simulink library "lib_controls2"  (Simulink 10.1)
settings: Solver=VariableStepAuto  StartTime=0.0  StopTime=10.0  RelTol=1e-3
undefined symbols (not defined in the file or in its folder): cs_charge_deplete_bool, cs_charge_pwr, cs_charge_trq, cs_fc_init_state, cs_hi_soc, cs_lo_soc, cs_max_pwr, cs_max_pwr_fall_rate, cs_max_pwr_rise_rate, cs_min_off_time, cs_min_pwr, cs_min_trq_frac, cs_pwr, cs_spd, ess_on, fc_map_spd, fc_max_trq, fc_on, fc_spd_scale, fc_trq_scale, gc_map_spd, gc_map_trq, gc_outpwr_map, gc_spd_scale, gc_trq_scale
settings Model: Creator=sateeshk  LastModifiedBy=sateeshk
settings Model: ModifiedComment=|
  | bjeanner -- Thu Dec 26 09:42:29 2002 -- Version 1.451
  | add three new parameters: allowing calcultion of equivallent ESS function with mean efficiency; plus plotting results parameter
settings Model: ModifiedHistory=|
  | bjeanner -- Thu Dec 26 09:42:29 2002 -- Version 1.451
  | add three new parameters: allowing calcultion of equivallent ESS function with mean efficiency; plus plotting results parameter
  | 
  | 
  | bjeanner -- Thu Dec 26 09:42:29 2002 -- Version 1.451
  | add three new parameters: allowing calcultion of equivallent ESS function with mean efficiency; plus plotting results parameter
  | 
  | 
  | bjeanner -- Thu Dec 12 14:52:52 2002 -- Version 1.450
  | 
  | 
  | bjeanner -- Tue Dec 10 14:49:05 2002 -- Version 1.449
  | 
  | 
  | bjeanner -- Tue Dec 10 13:14:31 2002 -- Version 1.448
  | 
  | 
  | bjeanner -- Tue Dec 10 11:50:56 2002 -- Version 1.447
  | 
  | 
  | bjeanner -- Tue Dec 10 11:41:01 2002 -- Version 1.446
  | 
  | 
  | bjeanner -- Tue Dec 10 11:30:40 2002 -- Version 1.445
  | 
  | 
  | bjeanner -- Tue Dec 10 11:29:40 2002 -- Version 1.444
  | 
  | 
  | bjeanner -- Tue Dec 10 11:10:40 2002 -- Version 1.443
  | 
  | 
  | bjeanner -- Tue Dec 10 10:31:25 2002 -- Version 1.442
  | 
  | 
  | bjeanner -- Tue Dec 10 10:30:04 2002 -- Version 1.441
  | 
  | 
  | bjeanner -- Tue Dec 10 10:29:36 2002 -- Version 1.440
  | 
  | 
  | bjeanner -- Tue Dec 10 10:23:30 2002 -- Version 1.439
  | 
  | 
  | bjeanner -- Tue Dec 10 09:20:40 2002 -- Version 1.438
  | 
  | 
  | bjeanner -- Tue Dec 10 09:16:26 2002 -- Version 1.437
  | Add the template for the configurable subsystem for the BD_FUELCELL control strategy.
  | Add the fuel cell adaptive control strategy
  | 
  | 
  | mokeefe -- Tue Aug 13 07:36:17 2002 -- Version 1.436
  | Making the model look "pretty"
  | 
  | mokeefe -- Tue Aug 13 07:35:11 2002 -- Version 1.435
  | changed <vc> conv cvt/cvt control to use "acc_mech_pwr_est" instead of "acc_mech_trq_est" as had been used previously (the required datum is the power and not the torque!)
  | 
  | ssprik -- Tue Apr 30 11:21:35 2002 -- Version 1.434
  | added user contributed par bal engine on  block
  | 
  | mokeefe -- Tue Apr 23 09:06:10 2002 -- Version 1.433
  | changed Insight electric assist control strategy <cs> DIRECT SPLIT/Hard Acceleration to prevent a divide by zero warning. Also added logic to prevent a torque request above the maximum achievable motor torque.
  | 
  | mokeefe -- Tue Apr 23 09:03:51 2002 -- Version 1.432
  | changed Insight electric assist control strategy <cs> DIRECT SPLIT/Hard Acceleration to prevent a divide by zero warning. Also added logic to prevent a torque request above the maximum achievable motor torque.
  | 
  | mokeefe -- Tue Apr 23 08:50:58 2002 -- Version 1.431
  | 
  | 
  | ssprik -- Thu Apr 18 14:34:50 2002 -- Version 1.430
  | 
  | 
  | ssprik -- Thu Apr 18 14:32:52 2002 -- Version 1.429
  | 
  | 
  | ssprik -- Thu Apr 18 14:06:57 2002 -- Version 1.428
  | 
  | 
  | ssprik -- Thu Apr 18 13:56:10 2002 -- Version 1.427
  | 
  | 
  | ssprik -- Thu Apr 18 13:46:32 2002 -- Version 1.426
  | 
  | 
  | kkelly -- Thu Apr 18 10:17:40 2002 -- Version 1.425
  | 
  | 
  | mokeefe -- Thu Apr 18 08:23:32 2002 -- Version 1.424
  | saving the model:
  | o "without the model browser open"
  | o with only top-level screen visible
  | o with "fit to view" enabled
  | o with "status bar" off and "toolbar" off
  | o with "prompt to update model history with each save" on
  | 
  | kkelly -- Wed Mar 27 14:57:12 2002 -- Version 1.423
  | 
  | 
  | kkelly -- Wed Mar 27 14:57:12 2002 -- Version 1.423
  | 
  | 
  | kkelly -- Wed Mar 27 14:50:41 2002 -- Version 1.422
  | 
  | 
  | kkelly -- Wed Mar 27 14:50:24 2002 -- Version 1.421
  | 
  | 
  | kkelly -- Wed Mar 27 14:26:31 2002 -- Version 1.420
  | 
  | 
  | kkelly -- Wed Mar 27 14:26:16 2002 -- Version 1.419
  | 
  | 
  | kkelly -- Wed Mar 27 14:25:54 2002 -- Version 1.418
  | 
  | 
  | kkelly -- Wed Mar 27 14:20:49 2002 -- Version 1.417
  | 
  | 
  | kkelly -- Wed Mar 27 14:18:25 2002 -- Version 1.416
  | 
  | 
  | kkelly -- Wed Mar 27 14:17:14 2002 -- Version 1.415
  | 
  | 
  | kkelly -- Wed Mar 27 14:09:18 2002 -- Version 1.414
  | 
  | 
  | kkelly -- Wed Mar 27 14:07:10 2002 -- Version 1.413
  | 
  | 
  | kkelly -- Wed Mar 27 14:04:42 2002 -- Version 1.412
  | 
  | 
  | kkelly -- Wed Mar 27 12:39:55 2002 -- Version 1.411
  | 
  | 
  | kkelly -- Wed Mar 27 12:39:35 2002 -- Version 1.410
  | 
  | 
  | kkelly -- Wed Mar 27 12:31:18 2002 -- Version 1.409
  | 
  | 
  | kkelly -- Wed Mar 27 12:12:25 2002 -- Version 1.408
  | 
  | 
  | kkelly -- Wed Mar 27 12:03:57 2002 -- Version 1.407
  | 
  | 
  | kkelly -- Wed Mar 27 12:03:11 2002 -- Version 1.406
  | Added logic to increase torque request for very hard acceleration
  | 
  | kkelly -- Wed Mar 27 11:51:32 2002 -- Version 1.405
  | Added logic to allow EM in 1st gear when torque request is high
  | 
  | kkelly -- Wed Mar 27 11:48:18 2002 -- Version 1.404
  | Added logic to allow EM at low speed with high torque request
  | 
  | kkelly -- Wed Mar 27 11:36:20 2002 -- Version 1.403
  | Added zero-torque request logic
  | 
  | kkelly -- Wed Mar 27 11:09:35 2002 -- Version 1.402
  | 
  | 
  | kkelly -- Wed Mar 27 11:07:39 2002 -- Version 1.401
  | 
  | 
  | kkelly -- Wed Mar 27 10:43:33 2002 -- Version 1.400
  | 
  | 
  | mokeefe -- Fri Mar 08 08:11:28 2002 -- Version 1.399
  | took all separate auxiliary load calculations out of the <vc> libraries. These will now use the lib_accessory goto tags (acc_mech_trq_est, acc_mech_pwr_est, acc_elec_pwr_est)
  | 
  | mokeefe -- Mon Jul 02 10:08:55 2001 -- Version 1.184
  | 
  | 
  | mokeefe -- Mon Jul 02 10:08:07 2001 -- Version 1.183
  | 
  | 
  | mokeefe -- Mon Jul 02 10:06:51 2001 -- Version 1.182
  | 
  | 
  | mokeefe -- Mon Jul 02 10:05:17 2001 -- Version 1.181
  | 
  | 
  | mokeefe -- Mon Jul 02 10:04:17 2001 -- Version 1.180
  | 
  | 
  | mokeefe -- Fri Jun 29 13:59:18 2001 -- Version 1.179
  | 
  | all <vc> blocks updated for use with variable cargo mass functionality (cargo mass by distance)--also, all <vc> top-level blocks have been "cleaned up" to look neat and organized. A sub-model library has been made and is the preferred way to do future development.
  | 
  | mokeefe -- Fri Jun 29 13:56:37 2001 -- Version 1.178
  | 
  | <vc> prius
  | 
  | mokeefe -- Fri Jun 29 13:46:29 2001 -- Version 1.177
  | 
  | 
  | mokeefe -- Fri Jun 29 13:40:43 2001 -- Version 1.176
  | 
  | 
  | mokeefe -- Fri Jun 29 13:39:38 2001 -- Version 1.175
  | 
  | <vc> series ("" "")
  | 
  | 
  | mokeefe -- Fri Jun 29 13:34:00 2001 -- Version 1.174
  | 
  | <vc> par Adaptive ("" "")
  | 
  | mokeefe -- Fri Jun 29 13:23:41 2001 -- Version 1.173
  | 
  | insight (ibid.)
  | 
  | 
  | mokeefe -- Fri Jun 29 13:15:22 2001 -- Version 1.172
  | 
  | <vc> par balanced--> veh_mass to veh_mass+veh_cargo_mass
  | 
  | 
  | mokeefe -- Fri Jun 29 13:05:39 2001 -- Version 1.171
  | 
  | 
  | mokeefe -- Fri Jun 29 12:10:12 2001 -- Version 1.170
  | 
  | finished veh_mass mods for the <vc> par cvt...
  | 
  | 
  | mokeefe -- Fri Jun 29 12:09:18 2001 -- Version 1.169
  | 
  | 
  | mokeefe -- Fri Jun 29 11:56:20 2001 -- Version 1.168
  | 
  | 
  | mokeefe -- Fri Jun 29 11:44:30 2001 -- Version 1.167
  | 
  | 
  | mokeefe -- Fri Jun 29 11:33:07 2001 -- Version 1.166
  | 
  | 
  | mokeefe -- Fri Jun 29 11:21:54 2001 -- Version 1.165
  | 
  | 
  | mokeefe -- Fri Jun 29 11:15:04 2001 -- Version 1.164
  | 
  | 
  | mokeefe -- Fri Jun 29 11:13:02 2001 -- Version 1.163
  | 
  | 
  | mokeefe -- Fri Jun 29 11:06:47 2001 -- Version 1.162
  | 
  | 
  | mokeefe -- Fri Jun 29 11:04:27 2001 -- Version 1.161
  | 
  | 
  | mokeefe -- Fri Jun 29 10:40:33 2001 -- Version 1.160
  | 
  | 
  | mokeefe -- Fri Jun 29 10:35:18 2001 -- Version 1.159
  | 
  | 
  | mokeefe -- Fri Jun 29 10:29:06 2001 -- Version 1.158
  | 
  | 
  | mokeefe -- Fri Jun 29 10:26:50 2001 -- Version 1.157
  | 
  | 
  | mokeefe -- Fri Jun 29 10:18:10 2001 -- Version 1.156
  | 
  | made traction control, front and rear brake controller, and braking strategy into "sub-libraries" for vehicle control
  | 
  | mokeefe -- Fri Jun 29 10:17:11 2001 -- Version 1.155
  | 
  | 
  | mokeefe -- Fri Jun 29 10:15:46 2001 -- Version 1.154
  | 
  | 
  | mokeefe -- Fri Jun 29 10:09:48 2001 -- Version 1.153
  | 
  | 
  | mokeefe -- Fri Jun 29 09:58:42 2001 -- Version 1.152
  | 
  | 
  | mokeefe -- Fri Jun 29 09:57:37 2001 -- Version 1.151
  | 
  | creating sub-components for vehicle control model (traction control)
  | 
  | mokeefe -- Fri Jun 29 09:21:23 2001 -- Version 1.150
  | 
  | 
  | mokeefe -- Fri Jun 29 09:19:46 2001 -- Version 1.149
  | 
  | 
  | mokeefe -- Fri Jun 29 09:09:49 2001 -- Version 1.148
  | 
  | 
  | mokeefe -- Fri Jun 29 08:32:46 2001 -- Version 1.147
  | 
  | 
  | mokeefe -- Fri Jun 29 08:29:03 2001 -- Version 1.146
  | 
  | replacing veh_mass with veh_mass plus veh_cargo_mass in <vc> conv auto Saber Custom
  | 
  | 
  | mokeefe -- Thu Jun 28 17:08:40 2001 -- Version 1.145
  | 
  | 
  | mokeefe -- Thu Jun 28 17:07:02 2001 -- Version 1.144
  | 
  | 
  | mokeefe -- Thu Jun 28 17:06:28 2001 -- Version 1.143
  | 
  | changes to the CVT controls to subsitute veh_mass + veh_cargo_mass for veh_mass
  | 
  | 
  | mokeefe -- Thu Jun 28 16:55:42 2001 -- Version 1.142
  | 
  | 
  | mokeefe -- Thu Jun 28 16:32:01 2001 -- Version 1.141
  | 
  | changing veh_mass to veh_mass plus veh_cargo_mass
  | 
  | 
  | mokeefe -- Thu Jun 28 16:21:30 2001 -- Version 1.140
  | 
  | replacing veh_mass with veh_mass + (cargo mass vs time)
  | 
  | mokeefe -- Thu Jun 28 14:12:51 2001 -- Version 1.139
  | 
  | replaced all 'veh_mass' references with a veh_mass plus a FROM block (originating from drive cycle) that gives variable cargo mass by time

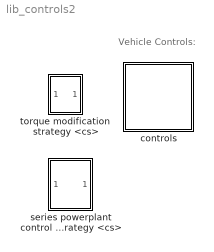
== system lib_controls2 ==
  note: Vehicle Controls:
  controls : Subsystem
  series powerplant control strategy <cs> : Subsystem  mask(Stand-Alone Series Powerplant Control Strategy Mask){generalName='cs', logPick=Log, initFileName={}, modCell={}, imgFileName='bdi_cs.jpg', DEBUG=OFF}
      mask prompts: generalName "General Name of this Component [char]"; logPick "Log Variables to Workspace?"; initFileName "Initialization File(s) [cell array of char]"; modCell "Modification Cell [2 column cell array of param and val]"; imgFileName "Icon image file name [char--evaluated]"
      mask init:
      | % initialization via m-file script
      | advSACompMaskInit;
      mask TypeOptions logPick: Don't Log | Log
      mask TypeOptions DEBUG: ON | OFF
      mask Display: image(imread(imgFileName))
  torque modification  strategy <cs> : Subsystem  mask(Stand-Alone Torque Modification Strategy Mask){generalName='tm', logPick=Log, initFileName={}, modCell={}, imgFileName='bdi_hybrid_cntrl.jpg', DEBUG=OFF}
      mask prompts: generalName "General Name of this Component [char]"; logPick "Log Variables to Workspace?"; initFileName "Initialization File(s) [cell array of char]"; modCell "Modification Cell [2 column cell array of param and val]"; imgFileName "Icon image file name [char--evaluated]"
      mask init:
      | % initialization via m-file script
      | advSACompMaskInit;
      mask TypeOptions logPick: Don't Log | Log
      mask TypeOptions DEBUG: ON | OFF
      mask Display: image(imread(imgFileName))

== system lib_controls2/controls ==
  Hybrid  Engine Torque Modification Strategy : Subsystem
      mask Display: image(imread('bdi_hybrid_cntrl.jpg'))

== system lib_controls2/series powerplant control strategy <cs> ==
  note: Series Powerplant Control Strategy
  power req'd by bus (W) : Inport
  Model and Interface : Subsystem
  power follower : Subsystem
      settings: OpenFcn=web(['file:\\\' which('Series.htm')]);
      mask Display: image(imread('doc_man.jpg'))
  thermostat : Subsystem
      settings: OpenFcn=web(['file:\\\' which('Series-therm.htm')]);
      mask Display: image(imread('doc_man.jpg'))
  "engine torque and speed (Nm), (rad/s)" : Outport  InitialOutput=0
  tag scope: csReqOut=global, csSensors=global
  wires:
  Model and Interface/2("engine torque and speed (Nm), (rad/s)") -> "engine torque and speed (Nm), (rad/s)"/1
  power req'd by bus (W)/1 -> Model and Interface/1(power req'd by bus (W))
  Model and Interface/1(req'd out) -> [csReqOut]
  [csControl] -> Model and Interface/2(control)
  Model and Interface/3(sensors) -> [csSensors]

== system lib_controls2/torque modification  strategy <cs> ==
  note: Torque Modification Strategy
  "original torque and speed req'd (Nm), (rad/s)" : Inport
  Block NOTES : Subsystem
      mask Display: disp('Block\nNOTES')
  help1 : Subsystem
      settings: OpenFcn=web(['file:\\\' which('cs_tips.htm')]);
      mask Display: image(imread('doc_man.jpg'))
  torque mod  model & interface : Subsystem
  "modified torque and speed req'd (Nm), (rad/s)" : Outport  InitialOutput=0
  tag scope: tmReqOut=global, tmSensors=global
  wires:
  torque mod  model & interface/3(sensors) -> [tmSensors]
  [tmControl] -> torque mod  model & interface/2(controls)
  "original torque and speed req'd (Nm), (rad/s)"/1 -> torque mod  model & interface/1(trq and spd output request)
  torque mod  model & interface/2(trq and spd input request) -> "modified torque and speed req'd (Nm), (rad/s)"/1
  torque mod  model & interface/1(requested output) -> [tmReqOut]

== system lib_controls2/controls/Hybrid  Engine Torque Modification Strategy ==
  Bus Creator : BusCreator  Inputs=3
  Bus Selector : BusSelector  OutputSignals=tm_spd_out_r
  Bus Selector1 : BusSelector  OutputSignals=SOC
  Bus Selector2 : BusSelector  OutputSignals=engine_on
  parallel auto hybrid torque control : Subsystem
  tag scope: tmControl=global
  wires:
  parallel auto hybrid torque control/1(tm_torqueMod) -> Bus Creator/1  "tm_torqueMod"
  parallel auto hybrid torque control/2(tm_torqueMin) -> Bus Creator/2  "tm_torqueMin"
  parallel auto hybrid torque control/3(tm_enable) -> Bus Creator/3  "tm_enable"
  Bus Creator/1 -> [tmControl]
  [tmReqOut] -> Bus Selector/1
  Bus Selector/1 -> parallel auto hybrid torque control/1(tm_spd_out_r)  "<tm_spd_out_r>"
  [essSensors] -> Bus Selector1/1
  Bus Selector1/1 -> parallel auto hybrid torque control/2(SOC)  "<SOC>"
  [fcControl] -> Bus Selector2/1
  Bus Selector2/1 -> parallel auto hybrid torque control/3(engine_on)  "<engine_on>"

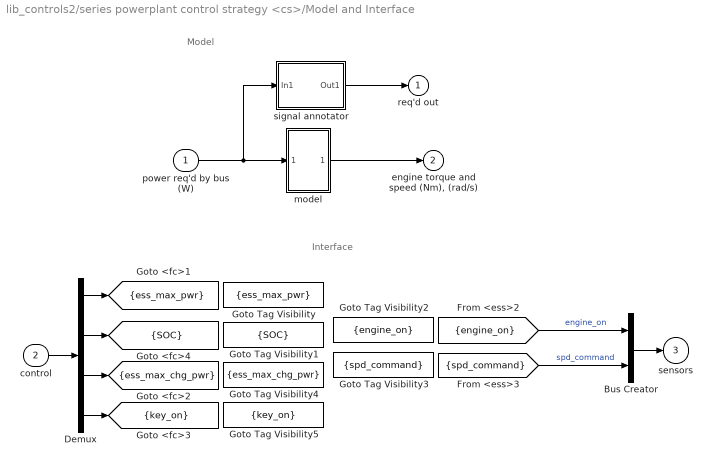
== system lib_controls2/series powerplant control strategy <cs>/Model and Interface ==
  note: Interface
  note: Model
  power req'd by bus (W) : Inport
  control : Inport  Port=2
  Bus Creator : BusCreator  Inputs=2
  Demux : Demux
  Goto Tag Visibility : GotoTagVisibility  GotoTag=ess_max_pwr
  Goto Tag Visibility1 : GotoTagVisibility  GotoTag=SOC
  Goto Tag Visibility2 : GotoTagVisibility  GotoTag=engine_on
  Goto Tag Visibility3 : GotoTagVisibility  GotoTag=spd_command
  Goto Tag Visibility4 : GotoTagVisibility  GotoTag=ess_max_chg_pwr
  Goto Tag Visibility5 : GotoTagVisibility  GotoTag=key_on
  model : Subsystem
  signal annotator : Subsystem
  req'd out : Outport  InitialOutput=0
  "engine torque and speed (Nm), (rad/s)" : Outport  Port=2  InitialOutput=0
  sensors : Outport  Port=3  InitialOutput=0
  tag scope: SOC=scoped, ess_max_chg_pwr=scoped, ess_max_pwr=scoped, key_on=scoped
  wires:
  model/1(Out1) -> "engine torque and speed (Nm), (rad/s)"/1
  power req'd by bus (W)/1 -> model/1(In1), signal annotator/1(In1)
  signal annotator/1(Out1) -> req'd out/1
  control/1 -> Demux/1
  Demux/1 -> [ess_max_pwr]
  Demux/2 -> [SOC]
  Demux/3 -> [ess_max_chg_pwr]
  Demux/4 -> [key_on]
  Bus Creator/1 -> sensors/1
  [engine_on] -> Bus Creator/1  "engine_on"
  [spd_command] -> Bus Creator/2  "spd_command"

== system lib_controls2/series powerplant control strategy <cs>/power follower ==

== system lib_controls2/series powerplant control strategy <cs>/thermostat ==

== system lib_controls2/torque modification  strategy <cs>/Block NOTES ==
  note: This model allows for increasing or decreasing of torque along a connection for purposes
      | of hybrid charging and control strategy.

== system lib_controls2/torque modification  strategy <cs>/help1 ==

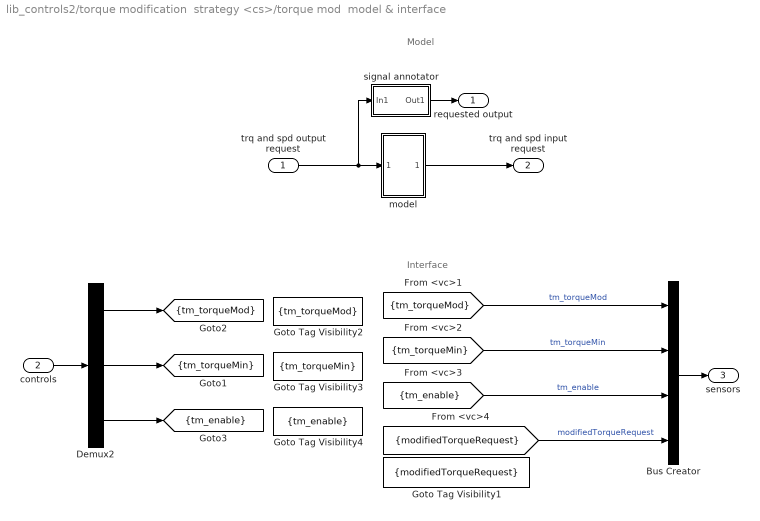
== system lib_controls2/torque modification  strategy <cs>/torque mod  model & interface ==
  note: Interface
  note: Model
  trq and spd output request : Inport
  controls : Inport  Port=2
  Bus Creator : BusCreator  Inputs=4
  Demux2 : Demux  Outputs=3
  Goto Tag Visibility1 : GotoTagVisibility  GotoTag=modifiedTorqueRequest
  Goto Tag Visibility2 : GotoTagVisibility  GotoTag=tm_torqueMod
  Goto Tag Visibility3 : GotoTagVisibility  GotoTag=tm_torqueMin
  Goto Tag Visibility4 : GotoTagVisibility  GotoTag=tm_enable
  model : Subsystem
  signal annotator : Subsystem
  requested output : Outport
  trq and spd input request : Outport  Port=2
  sensors : Outport  Port=3
  tag scope: tm_enable=scoped, tm_torqueMin=scoped, tm_torqueMod=scoped
  wires:
  signal annotator/1(Out1) -> requested output/1
  model/1(T,w modified) -> trq and spd input request/1
  trq and spd output request/1 -> signal annotator/1(In1), model/1("T, w original")
  Demux2/1 -> [tm_torqueMod]
  controls/1 -> Demux2/1
  Bus Creator/1 -> sensors/1
  [tm_torqueMod] -> Bus Creator/1  "tm_torqueMod"
  Demux2/2 -> [tm_torqueMin]
  Demux2/3 -> [tm_enable]
  [tm_torqueMin] -> Bus Creator/2  "tm_torqueMin"
  [tm_enable] -> Bus Creator/3  "tm_enable"
  [modifiedTorqueRequest] -> Bus Creator/4  "modifiedTorqueRequest"

== system lib_controls2/controls/Hybrid  Engine Torque Modification Strategy/parallel auto hybrid torque control ==
  tm_spd_out_r : Inport
  SOC : Inport  Port=2
  engine_on : Inport  Port=3
  chg trq req'd (Nm) : Subsystem
  minimum trq (Nm) : Subsystem
  tm_torqueMod : Outport
  tm_torqueMin : Outport  Port=2
  tm_enable : Outport  Port=3
  wires:
  tm_spd_out_r/1 -> minimum trq (Nm)/1("spd req'd in (N*m, rad/s)")
  SOC/1 -> minimum trq (Nm)/2(SOC), chg trq req'd (Nm)/1(SOC)
  minimum trq (Nm)/1(minimum trq (N*m)) -> tm_torqueMin/1
  engine_on/1 -> tm_enable/1
  chg trq req'd (Nm)/1(add'l trq req'd (Nm)) -> tm_torqueMod/1

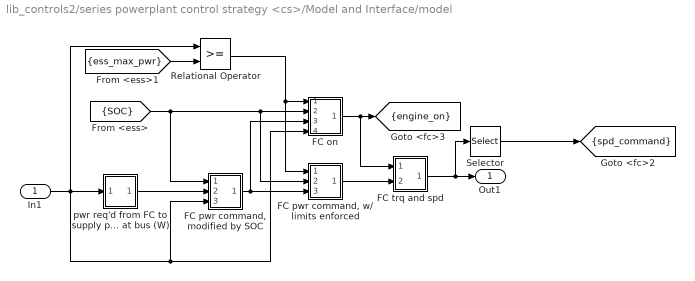
== system lib_controls2/series powerplant control strategy <cs>/Model and Interface/model ==
  In1 : Inport
  FC on : Subsystem
  "FC pwr command, modified by SOC" : Subsystem
  "FC pwr command, w/ limits enforced" : Subsystem
  FC trq and spd : Subsystem
  Relational Operator : RelationalOperator  RndMeth=Nearest  InputSameDT=on
  Selector : Selector  InputPortWidth=2  IndexOptions=Index vector (dialog)  Indices=2  OutputSizes=1
  pwr req'd from FC to supply pwr req'd at bus (W) : Subsystem
  Out1 : Outport
  tag scope: engine_on=scoped, spd_command=scoped
  wires:
  [SOC] -> "FC pwr command, modified by SOC"/1(SOC), "FC pwr command, w/ limits enforced"/2(SOC), FC on/2(SOC)
  "FC pwr command, modified by SOC"/1(pwr command modifed for SOC (W)) -> FC on/3(FC pwr command), "FC pwr command, w/ limits enforced"/3(FC pwr command)
  pwr req'd from FC to supply pwr req'd at bus (W)/1(pwr req'd of FC (W)) -> "FC pwr command, modified by SOC"/2(raw pwr command (W))
  Relational Operator/1 -> "FC pwr command, w/ limits enforced"/1(ess max pwr would be insufficient), FC on/1(ess max pwr would be insufficient)
  [ess_max_pwr] -> Relational Operator/2
  In1/1 -> pwr req'd from FC to supply pwr req'd at bus (W)/1(power req'd by bus (W)), Relational Operator/1, "FC pwr command, modified by SOC"/3(pwr req'd at bus (W)), FC on/4(bus pwr req)
  FC on/1(FC on) -> FC trq and spd/1(FC on), [engine_on]
  "FC pwr command, w/ limits enforced"/1(limited FC pwr command (W)) -> FC trq and spd/2(power req'd by FC (W))
  FC trq and spd/1("engine torque and speed (Nm), (rad/s)") -> Selector/1, Out1/1
  Selector/1 -> [spd_command]

== system lib_controls2/series powerplant control strategy <cs>/Model and Interface/signal annotator ==
  In1 : Inport
  Out1 : Outport
  wires:
  In1/1 -> Out1/1  "power requirement"

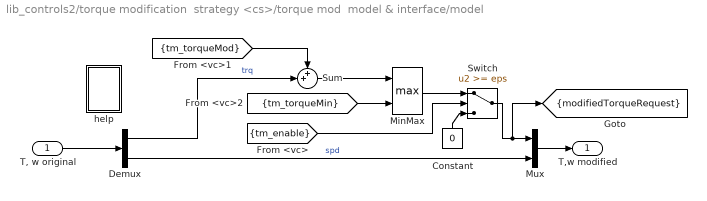
== system lib_controls2/torque modification  strategy <cs>/torque mod  model & interface/model ==
  "T, w original" : Inport
  Constant : Constant  Value=0
  Demux : Demux  Outputs=2
  MinMax : MinMax  Function=max  Inputs=2
  Mux : Mux  Inputs=2
  Sum : Sum  Inputs=++|  SaturateOnIntegerOverflow=on
  Switch : Switch  Threshold=eps  SaturateOnIntegerOverflow=on  InputSameDT=on
  help : Subsystem
      settings: OpenFcn=web(['file:\\\' which('Parallel.htm')])
      mask Display: image(imread('doc_man.jpg'))
  T,w modified : Outport
  tag scope: modifiedTorqueRequest=scoped
  wires:
  [tm_torqueMin] -> MinMax/2
  Switch/1 -> Mux/1, [modifiedTorqueRequest]
  Constant/1 -> Switch/3
  MinMax/1 -> Switch/1
  Sum/1 -> MinMax/1
  [tm_torqueMod] -> Sum/1
  [tm_enable] -> Switch/2
  Mux/1 -> T,w modified/1
  "T, w original"/1 -> Demux/1
  Demux/1 -> Sum/2  "trq"
  Demux/2 -> Mux/2  "spd"

== system lib_controls2/torque modification  strategy <cs>/torque mod  model & interface/signal annotator ==
  In1 : Inport
  Demux : Demux  Outputs=2
  Mux : Mux  Inputs=2
  Out1 : Outport
  wires:
  Mux/1 -> Out1/1
  Demux/2 -> Mux/2  "tm_spd_out_r"
  Demux/1 -> Mux/1  "tm_trq_out_r"
  In1/1 -> Demux/1

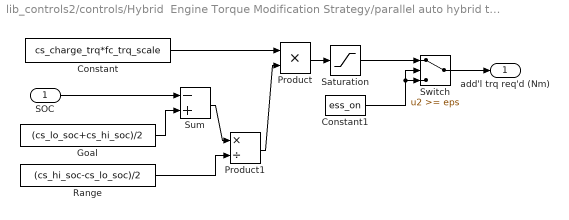
== system lib_controls2/controls/Hybrid  Engine Torque Modification Strategy/parallel auto hybrid torque control/chg trq req'd (Nm) ==
  SOC : Inport
  Constant : Constant  Value=cs_charge_trq*fc_trq_scale
  Constant1 : Constant  Value=ess_on
  Goal : Constant  Value=(cs_lo_soc+cs_hi_soc)/2
  Product : Product  SaturateOnIntegerOverflow=on
  Product1 : Product  Inputs=*/  SaturateOnIntegerOverflow=on
  Range : Constant  Value=(cs_hi_soc-cs_lo_soc)/2
  Saturation : Saturate  UpperLimit=inf  LowerLimit=-inf
  Sum : Sum  Inputs=-+  SaturateOnIntegerOverflow=on
  Switch : Switch  Threshold=eps  SaturateOnIntegerOverflow=on  InputSameDT=on
  add'l trq req'd (Nm) : Outport
  wires:
  Constant1/1 -> Switch/3, Switch/2
  Switch/1 -> add'l trq req'd (Nm)/1
  Saturation/1 -> Switch/1
  Goal/1 -> Sum/2
  Range/1 -> Product1/2
  Sum/1 -> Product1/1
  Product1/1 -> Product/2
  Constant/1 -> Product/1
  Product/1 -> Saturation/1
  SOC/1 -> Sum/1

== system lib_controls2/controls/Hybrid  Engine Torque Modification Strategy/parallel auto hybrid torque control/minimum trq (Nm) ==
  "spd req'd in (N*m, rad/s)" : Inport
  SOC : Inport  Port=2
  (--) : Constant  Value=cs_lo_soc
  Constant : Constant  Value=0
  Gain : Gain  Gain=cs_min_trq_frac  SaturateOnIntegerOverflow=on
  Relational Operator2 : RelationalOperator  Operator=<  RndMeth=Nearest  InputSameDT=on
  Switch : Switch  Threshold=eps  SaturateOnIntegerOverflow=on  InputSameDT=on
  max_torque lookup : Lookup  InputValues=fc_map_spd  Table=fc_max_trq*fc_trq_scale  SaturateOnIntegerOverflow=on
  minimum trq (N*m) : Outport
  wires:
  Gain/1 -> Switch/1
  max_torque lookup/1 -> Gain/1
  "spd req'd in (N*m, rad/s)"/1 -> max_torque lookup/1
  Constant/1 -> Switch/3
  Switch/1 -> minimum trq (N*m)/1
  Relational Operator2/1 -> Switch/2
  (--)/1 -> Relational Operator2/2
  SOC/1 -> Relational Operator2/1

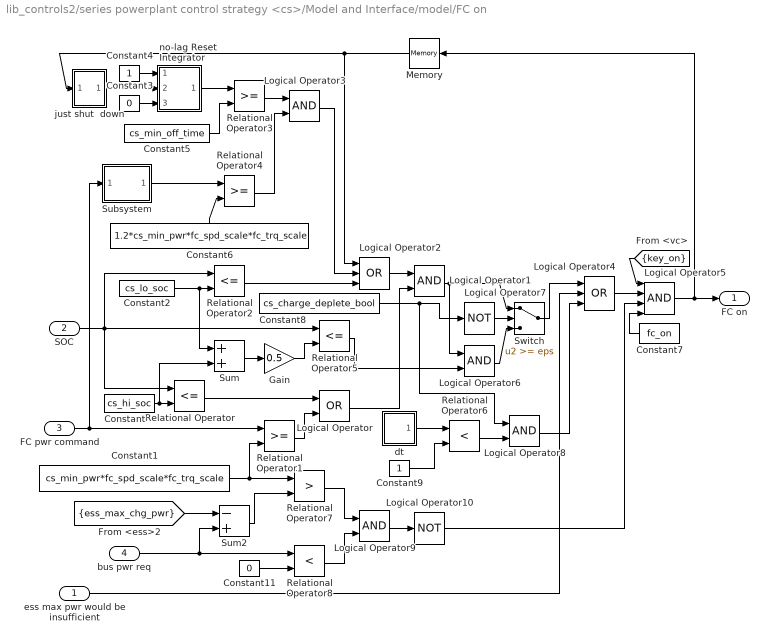
== system lib_controls2/series powerplant control strategy <cs>/Model and Interface/model/FC on ==
  ess max pwr would be insufficient : Inport
  SOC : Inport  Port=2
  FC pwr command : Inport  Port=3
  bus pwr req : Inport  Port=4
  Constant : Constant  Value=cs_hi_soc
  Constant1 : Constant  Value=cs_min_pwr*fc_spd_scale*fc_trq_scale
  Constant11 : Constant  Value=0
  Constant2 : Constant  Value=cs_lo_soc
  Constant3 : Constant  Value=0
  Constant4 : Constant
  Constant5 : Constant  Value=cs_min_off_time
  Constant6 : Constant  Value=1.2*cs_min_pwr*fc_spd_scale*fc_trq_scale
  Constant7 : Constant  Value=fc_on
  Constant8 : Constant  Value=cs_charge_deplete_bool
  Constant9 : Constant
  Gain : Gain  Gain=0.5  SaturateOnIntegerOverflow=on
  Logical Operator : Logic  Operator=OR
  Logical Operator{1,3,6,8..9} (5 alike) : Logic
  Logical Operator10 : Logic  Operator=NOT
  Logical Operator2 : Logic  Operator=OR  Inputs=3
  Logical Operator4 : Logic  Operator=OR  Inputs=3
  Logical Operator5 : Logic  Inputs=4
  Logical Operator7 : Logic  Operator=NOT  Inputs=1
  Memory : Memory  InitialCondition=cs_fc_init_state
  Relational Operator : RelationalOperator  Operator=<=  RndMeth=Nearest  InputSameDT=on
  Relational Operator1 : RelationalOperator  RndMeth=Nearest  InputSameDT=on
  Relational Operator2 : RelationalOperator  Operator=<=  RndMeth=Nearest  InputSameDT=on
  Relational Operator3 : RelationalOperator  RndMeth=Nearest  InputSameDT=on
  Relational Operator4 : RelationalOperator  RndMeth=Nearest  InputSameDT=on
  Relational Operator5 : RelationalOperator  Operator=<=  RndMeth=Nearest  InputSameDT=on
  Relational Operator6 : RelationalOperator  Operator=<  RndMeth=Nearest  InputSameDT=on
  Relational Operator7 : RelationalOperator  Operator=>  RndMeth=Nearest  InputSameDT=on
  Relational Operator8 : RelationalOperator  Operator=<  RndMeth=Nearest  InputSameDT=on
  Subsystem : Subsystem  mask(Running Average){n=5}
      mask prompts: n "Averaging Time (s)"
      mask help: Running Average
      mask Help: Output is the average of the last (Averaging Time) seconds of input.
      mask Display: disp('Running\nAverage')
  Sum : Sum  SaturateOnIntegerOverflow=on
  Sum2 : Sum  Inputs=-+  SaturateOnIntegerOverflow=on
  Switch : Switch  Threshold=eps  SaturateOnIntegerOverflow=on  InputSameDT=on
  dt : Subsystem
  just shut  down : Subsystem
  no-lag Reset Integrator : Subsystem  mask(No-lag Reset Integrator){initval=0}
      mask prompts: initval "Initial Value"
      mask help: No-lag Reset Integrator
      mask Help: Integrates first input using Euler technique.\nAt the time step that input 2 <> zero,\noutput is reset to input 3.
      mask Display: disp('1/s\nw/ reset\nno lag')
  FC on : Outport
  wires:
  Relational Operator6/1 -> Logical Operator8/2
  Constant9/1 -> Relational Operator6/2
  dt/1(out_1) -> Relational Operator6/1
  Logical Operator8/1 -> Logical Operator4/3
  Constant8/1 -> Logical Operator8/1, Logical Operator7/1
  Switch/1 -> Logical Operator4/1
  Logical Operator1/1 -> Logical Operator6/1, Switch/1
  Logical Operator6/1 -> Switch/3
  Logical Operator7/1 -> Switch/2
  Gain/1 -> Relational Operator5/2
  Sum/1 -> Gain/1
  Constant/1 -> Sum/2, Relational Operator/2
  Constant2/1 -> Sum/1, Relational Operator2/2
  Memory/1 -> just shut  down/1(state), Logical Operator2/1
  Constant5/1 -> Relational Operator3/2
  Relational Operator3/1 -> Logical Operator3/1
  no-lag Reset Integrator/1(out_1) -> Relational Operator3/1
  just shut  down/1(trigger) -> no-lag Reset Integrator/2(in_2)
  Constant3/1 -> no-lag Reset Integrator/3(in_3)
  Constant4/1 -> no-lag Reset Integrator/1(in_1)
  Constant6/1 -> Relational Operator4/2
  Relational Operator4/1 -> Logical Operator3/2
  Subsystem/1(out_1) -> Relational Operator4/1
  Logical Operator3/1 -> Logical Operator2/2
  Logical Operator2/1 -> Logical Operator1/1
  SOC/1 -> Relational Operator5/1, Relational Operator/1, Relational Operator2/1
  Relational Operator1/1 -> Logical Operator/2
  FC pwr command/1 -> Relational Operator1/1, Subsystem/1(in_1)
  ess max pwr would be insufficient/1 -> Logical Operator4/2
  Relational Operator5/1 -> Logical Operator6/2
  Relational Operator2/1 -> Logical Operator2/3
  Relational Operator/1 -> Logical Operator/1
  Constant11/1 -> Relational Operator8/2
  [ess_max_chg_pwr] -> Sum2/1
  bus pwr req/1 -> Relational Operator8/1, Sum2/2
  Sum2/1 -> Relational Operator7/2
  Logical Operator/1 -> Logical Operator1/2
  Logical Operator9/1 -> Logical Operator10/1
  Logical Operator4/1 -> Logical Operator5/2
  Logical Operator5/1 -> FC on/1, Memory/1
  [key_on] -> Logical Operator5/1
  Constant7/1 -> Logical Operator5/4
  Logical Operator10/1 -> Logical Operator5/3
  Relational Operator7/1 -> Logical Operator9/1
  Relational Operator8/1 -> Logical Operator9/2
  Constant1/1 -> Relational Operator1/2, Relational Operator7/1

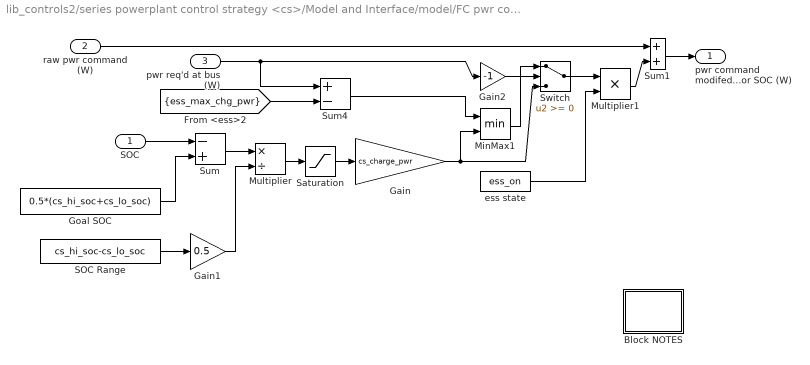
== system lib_controls2/series powerplant control strategy <cs>/Model and Interface/model/FC pwr command, modified by SOC ==
  SOC : Inport
  raw pwr command (W) : Inport  Port=2
  pwr req'd at bus (W) : Inport  Port=3
  Block NOTES : Subsystem
      mask Display: disp('Block\nNOTES')
  Gain : Gain  Gain=cs_charge_pwr  SaturateOnIntegerOverflow=on
  Gain1 : Gain  Gain=0.5  SaturateOnIntegerOverflow=on
  Gain2 : Gain  Gain=-1  SaturateOnIntegerOverflow=on
  Goal SOC : Constant  Value=0.5*(cs_hi_soc+cs_lo_soc)
  MinMax1 : MinMax  Inputs=2
  Multiplier : Product  Inputs=*/  SaturateOnIntegerOverflow=on
  Multiplier1 : Product  SaturateOnIntegerOverflow=on
  SOC Range : Constant  Value=cs_hi_soc-cs_lo_soc
  Saturation : Saturate  UpperLimit=1  LowerLimit=-1
  Sum : Sum  Inputs=-+  SaturateOnIntegerOverflow=on
  Sum1 : Sum  SaturateOnIntegerOverflow=on
  Sum4 : Sum  Inputs=+-  SaturateOnIntegerOverflow=on
  Switch : Switch  SaturateOnIntegerOverflow=on  InputSameDT=on
  ess state : Constant  Value=ess_on
  pwr command modifed for SOC (W) : Outport
  wires:
  ess state/1 -> Multiplier1/2
  Multiplier1/1 -> Sum1/2
  Switch/1 -> Multiplier1/1
  Sum1/1 -> pwr command modifed for SOC (W)/1
  SOC/1 -> Sum/1
  Goal SOC/1 -> Sum/2
  SOC Range/1 -> Gain1/1
  Multiplier/1 -> Saturation/1
  Sum/1 -> Multiplier/1
  Saturation/1 -> Gain/1
  Gain1/1 -> Multiplier/2
  MinMax1/1 -> Switch/1
  Gain/1 -> MinMax1/2, Switch/3
  Gain2/1 -> Switch/2
  raw pwr command (W)/1 -> Sum1/1
  pwr req'd at bus (W)/1 -> Sum4/1, Gain2/1
  [ess_max_chg_pwr] -> Sum4/2
  Sum4/1 -> MinMax1/1

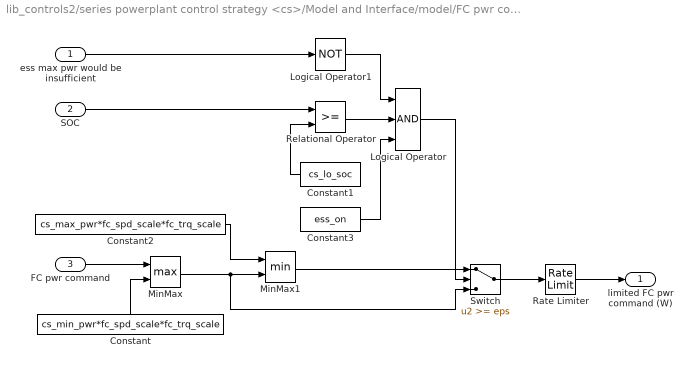
== system lib_controls2/series powerplant control strategy <cs>/Model and Interface/model/FC pwr command, w/ limits enforced ==
  ess max pwr would be insufficient : Inport
  SOC : Inport  Port=2
  FC pwr command : Inport  Port=3
  Constant : Constant  Value=cs_min_pwr*fc_spd_scale*fc_trq_scale
  Constant1 : Constant  Value=cs_lo_soc
  Constant2 : Constant  Value=cs_max_pwr*fc_spd_scale*fc_trq_scale
  Constant3 : Constant  Value=ess_on
  Logical Operator : Logic  Inputs=3
  Logical Operator1 : Logic  Operator=NOT  Inputs=1
  MinMax : MinMax  Function=max  Inputs=2
  MinMax1 : MinMax  Inputs=2
  Rate Limiter : RateLimiter  RisingSlewLimit=cs_max_pwr_rise_rate*fc_spd_scale*fc_trq_scale  FallingSlewLimit=cs_max_pwr_fall_rate*fc_spd_scale*fc_trq_scale
  Relational Operator : RelationalOperator  RndMeth=Nearest  InputSameDT=on
  Switch : Switch  Threshold=eps  SaturateOnIntegerOverflow=on  InputSameDT=on
  limited FC pwr command (W) : Outport
  wires:
  Constant3/1 -> Logical Operator/3
  Constant2/1 -> MinMax1/1
  MinMax1/1 -> Switch/1
  Switch/1 -> Rate Limiter/1
  Rate Limiter/1 -> limited FC pwr command (W)/1
  Constant1/1 -> Relational Operator/2
  Logical Operator/1 -> Switch/2
  Constant/1 -> MinMax/2
  MinMax/1 -> MinMax1/2, Switch/3
  FC pwr command/1 -> MinMax/1
  SOC/1 -> Relational Operator/1
  Relational Operator/1 -> Logical Operator/2
  Logical Operator1/1 -> Logical Operator/1
  ess max pwr would be insufficient/1 -> Logical Operator1/1

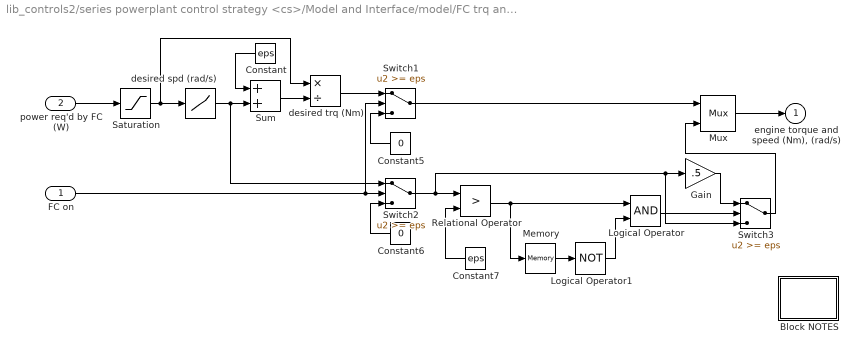
== system lib_controls2/series powerplant control strategy <cs>/Model and Interface/model/FC trq and spd ==
  FC on : Inport
  power req'd by FC (W) : Inport  Port=2
  Block NOTES : Subsystem
      mask Display: disp('Block\nNOTES')
  Constant : Constant  Value=eps
  Constant5 : Constant  Value=0
  Constant6 : Constant  Value=0
  Constant7 : Constant  Value=eps
  Gain : Gain  Gain=.5  SaturateOnIntegerOverflow=on
  Logical Operator : Logic
  Logical Operator1 : Logic  Operator=NOT  Inputs=1
  Memory : Memory
  Mux : Mux  Inputs=2
  Relational Operator : RelationalOperator  Operator=>  RndMeth=Nearest  InputSameDT=on
  Saturation : Saturate  UpperLimit=max(cs_pwr)  LowerLimit=min(cs_pwr)
  Sum : Sum  SaturateOnIntegerOverflow=on
  Switch1 : Switch  Threshold=eps  SaturateOnIntegerOverflow=on  InputSameDT=on
  Switch2 : Switch  Threshold=eps  SaturateOnIntegerOverflow=on  InputSameDT=on
  Switch3 : Switch  Threshold=eps  SaturateOnIntegerOverflow=on  InputSameDT=on
  desired spd (rad/s) : Lookup  InputValues=cs_pwr  Table=cs_spd  SaturateOnIntegerOverflow=on
  desired trq (Nm) : Product  Inputs=*/  SaturateOnIntegerOverflow=on
  "engine torque and speed (Nm), (rad/s)" : Outport  InitialOutput=0
  wires:
  Sum/1 -> desired trq (Nm)/2
  desired trq (Nm)/1 -> Switch1/1
  Constant/1 -> Sum/1
  power req'd by FC (W)/1 -> Saturation/1
  Saturation/1 -> desired spd (rad/s)/1, desired trq (Nm)/1
  Constant5/1 -> Switch1/3
  Constant6/1 -> Switch2/3
  desired spd (rad/s)/1 -> Sum/2, Switch2/1
  FC on/1 -> Switch1/2, Switch2/2
  Mux/1 -> "engine torque and speed (Nm), (rad/s)"/1
  Switch1/1 -> Mux/1
  Logical Operator/1 -> Switch3/2
  Constant7/1 -> Relational Operator/2
  Memory/1 -> Logical Operator1/1
  Relational Operator/1 -> Logical Operator/1, Memory/1
  Logical Operator1/1 -> Logical Operator/2
  Switch2/1 -> Relational Operator/1, Gain/1, Switch3/3
  Gain/1 -> Switch3/1
  Switch3/1 -> Mux/2

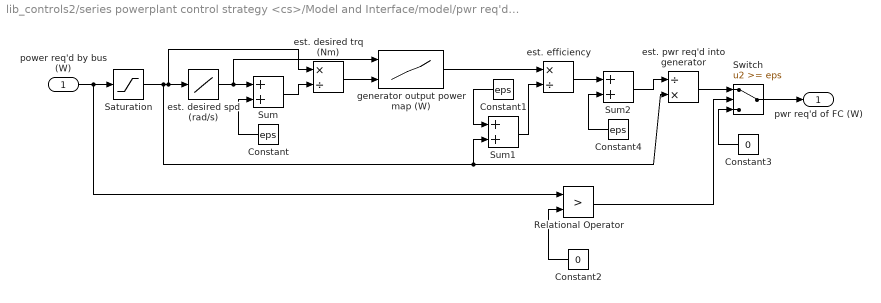
== system lib_controls2/series powerplant control strategy <cs>/Model and Interface/model/pwr req'd from FC to supply pwr req'd at bus (W) ==
  power req'd by bus (W) : Inport
  Constant : Constant  Value=eps
  Constant1 : Constant  Value=eps
  Constant2 : Constant  Value=0
  Constant3 : Constant  Value=0
  Constant4 : Constant  Value=eps
  Relational Operator : RelationalOperator  Operator=>  RndMeth=Nearest  InputSameDT=on
  Saturation : Saturate  UpperLimit=max(cs_pwr)  LowerLimit=min(cs_pwr)
  Sum : Sum  SaturateOnIntegerOverflow=on
  Sum1 : Sum  SaturateOnIntegerOverflow=on
  Sum2 : Sum  SaturateOnIntegerOverflow=on
  Switch : Switch  Threshold=eps  SaturateOnIntegerOverflow=on  InputSameDT=on
  est. efficiency : Product  Inputs=*/  SaturateOnIntegerOverflow=on
  est. desired spd (rad/s) : Lookup  InputValues=cs_pwr  Table=cs_spd  SaturateOnIntegerOverflow=on
  est. desired trq (Nm) : Product  Inputs=*/  SaturateOnIntegerOverflow=on
  est. pwr req'd into generator : Product  Inputs=/*  SaturateOnIntegerOverflow=on
  generator output power map (W) : Lookup2D  RowIndex=gc_map_spd*gc_spd_scale  ColumnIndex=gc_map_trq*gc_trq_scale  Table=gc_outpwr_map*gc_spd_scale*gc_trq_scale  SaturateOnIntegerOverflow=on  InputSameDT=on
  pwr req'd of FC (W) : Outport
  wires:
  Constant4/1 -> Sum2/2
  Sum2/1 -> est. pwr req'd into generator/1
  est. efficiency/1 -> Sum2/1
  est. pwr req'd into generator/1 -> Switch/1
  Switch/1 -> pwr req'd of FC (W)/1
  Relational Operator/1 -> Switch/2
  Constant3/1 -> Switch/3
  Sum/1 -> est. desired trq (Nm)/2
  Constant/1 -> Sum/2
  est. desired trq (Nm)/1 -> generator output power map (W)/2
  est. desired spd (rad/s)/1 -> Sum/1, generator output power map (W)/1
  Saturation/1 -> est. desired spd (rad/s)/1, est. desired trq (Nm)/1, est. pwr req'd into generator/2, Sum1/2
  generator output power map (W)/1 -> est. efficiency/1
  Sum1/1 -> est. efficiency/2
  Constant1/1 -> Sum1/1
  Constant2/1 -> Relational Operator/2
  power req'd by bus (W)/1 -> Saturation/1, Relational Operator/1

== system lib_controls2/torque modification  strategy <cs>/torque mod  model & interface/model/help ==

== system lib_controls2/series powerplant control strategy <cs>/Model and Interface/model/FC on/Subsystem ==
  in_1 : Inport
  Constant1 : Constant  Value=n
  Integrator : Integrator
  Product : Product  Inputs=*/  SaturateOnIntegerOverflow=on
  Sum : Sum  Inputs=+-  SaturateOnIntegerOverflow=on
  Transport Delay : TransportDelay  DelayTime=n
  out_1 : Outport  InitialOutput=0
  wires:
  Constant1/1 -> Product/2
  Product/1 -> out_1/1
  in_1/1 -> Integrator/1
  Sum/1 -> Product/1
  Transport Delay/1 -> Sum/2
  Integrator/1 -> Transport Delay/1, Sum/1

== system lib_controls2/series powerplant control strategy <cs>/Model and Interface/model/FC on/dt ==
  Clock : Clock
  Memory1 : Memory  InitialCondition=-1
  Sum1 : Sum  Inputs=+-  SaturateOnIntegerOverflow=on
  out_1 : Outport  InitialOutput=0
  wires:
  Sum1/1 -> out_1/1
  Memory1/1 -> Sum1/2
  Clock/1 -> Memory1/1, Sum1/1

== system lib_controls2/series powerplant control strategy <cs>/Model and Interface/model/FC on/just shut  down ==
  state : Inport
  Logical Operator : Logic
  Logical Operator1 : Logic  Operator=NOT  Inputs=1
  Memory1 : Memory  InitialCondition=1
  trigger : Outport  InitialOutput=0
  wires:
  Logical Operator/1 -> trigger/1
  Memory1/1 -> Logical Operator/2
  state/1 -> Memory1/1, Logical Operator1/1
  Logical Operator1/1 -> Logical Operator/1

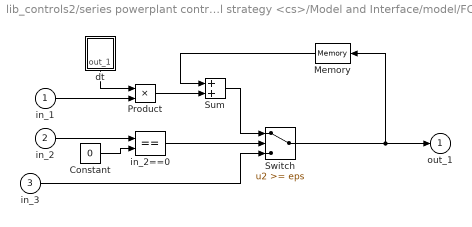
== system lib_controls2/series powerplant control strategy <cs>/Model and Interface/model/FC on/no-lag Reset Integrator ==
  in_1 : Inport
  in_2 : Inport  Port=2
  in_3 : Inport  Port=3
  Constant : Constant  Value=0
  Memory : Memory  InitialCondition=initval
  Product : Product  SaturateOnIntegerOverflow=on
  Sum : Sum  SaturateOnIntegerOverflow=on
  Switch : Switch  Threshold=eps  SaturateOnIntegerOverflow=on  InputSameDT=on
  dt : Subsystem
  in_2==0 : RelationalOperator  Operator===  RndMeth=Nearest  InputSameDT=on
  out_1 : Outport  InitialOutput=0
  wires:
  Constant/1 -> in_2==0/2
  in_2==0/1 -> Switch/2
  Switch/1 -> Memory/1, out_1/1
  Sum/1 -> Switch/1
  Memory/1 -> Sum/1
  Product/1 -> Sum/2
  dt/1(out_1) -> Product/1
  in_1/1 -> Product/2
  in_2/1 -> in_2==0/1
  in_3/1 -> Switch/3

== system lib_controls2/series powerplant control strategy <cs>/Model and Interface/model/FC pwr command, modified by SOC/Block NOTES ==
  note: 1/5/98/98:tm  Modified calculation of additional power required to maintain goal SOC
      | (SOC_goal - SOC_actual) / (0.5*SOC_range) * cs_charge_pwr
      | therefore when
      | actual_SOC=cs_lo_soc ==> 1.0  *cs_charge_pwr
      | actual_SOC=goal_SOC ==> 0.0  *cs_charge_pwr
      | actual_SOC=cs_hi_soc ==> -1.0 * cs_charge_pwr
      |
      | 2/6/01:tm added if battery disabled - do not modify request
  note: This block determines the additional power required of the fuel convertor
      |  to maintian an SOC equal to the average of cs_hi_soc and cs_lo_soc.

== system lib_controls2/series powerplant control strategy <cs>/Model and Interface/model/FC trq and spd/Block NOTES ==
  note: This block determines the required fuel converter torque and speed from the
      | required power using a vector usually representing the locus of best efficiency
      | or lowest emissions points in the map.  The speed request is cut in half if it is
      | nonzero and preceded by a zero speed request to account for the fact that all
      | ADVISOR's drivetrain components deal in speeds averaged over the time step.
      | A speed command here of 1/2 of max. engine speed means that the AVERAGE
      | engine speed required is 1/2 of max.  If the previous speed was zero, that means
      | that the speed at the end of the current time step must be equal to max. engine
      | speed.

== system lib_controls2/series powerplant control strategy <cs>/Model and Interface/model/FC on/no-lag Reset Integrator/dt ==
  Clock : Clock
  Memory1 : Memory  InitialCondition=-1
  Sum1 : Sum  Inputs=+-  SaturateOnIntegerOverflow=on
  out_1 : Outport  InitialOutput=0
  wires:
  Sum1/1 -> out_1/1
  Memory1/1 -> Sum1/2
  Clock/1 -> Memory1/1, Sum1/1
